simulink model "Performance_Model_0_0_1"  (R2014a)
settings: Solver=ode45  StartTime=0.0  StopTime=10.0  RelTol=1e-3
libraries: rocket_angular_flight_library x1, rocket_data_library x1, rocket_drag_library x1, rocket_isa_model_library x1, rocket_vertical_flight_library x1
settings Model: Creator=scorpii  LastModifiedBy=scorpii

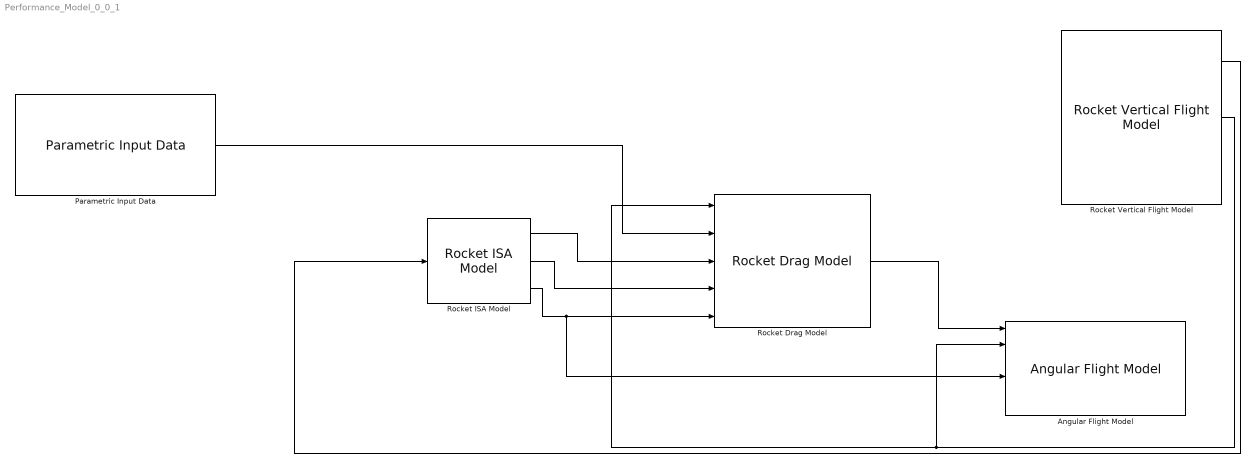
== system Performance_Model_0_0_1 ==
  Angular Flight Model : rocket_angular_flight_library/Angular Flight Model
  Parametric Input Data : rocket_data_library/Parametric Input Data
  Rocket Drag Model : rocket_drag_library/Rocket Drag Model
  Rocket ISA Model : rocket_isa_model_library/Rocket ISA Model
  Rocket Vertical Flight Model : rocket_vertical_flight_library/Rocket Vertical Flight Model
  wires:
  Parametric Input Data/1 -> Rocket Drag Model/2
  Rocket ISA Model/1 -> Rocket Drag Model/3
  Rocket ISA Model/2 -> Rocket Drag Model/4
  Rocket ISA Model/3 -> Angular Flight Model/4, Rocket Drag Model/5
  Rocket Vertical Flight Model/1 -> Rocket ISA Model/1
  Rocket Vertical Flight Model/2 -> Angular Flight Model/2, Rocket Drag Model/1
  Rocket Drag Model/1 -> Angular Flight Model/1
